simulink library "scp"  (R2021b)
settings: Solver=VariableStepAuto  StartTime=0.0  StopTime=10.0  RelTol=1e-3
undefined symbols (not defined in the file or in its folder): FALSE, KSCP_DelayECBAMandECDT_s, KSCP_DelayECDTandECDT_s, KSCP_DelayECDTandRCBAM_s, KSCP_DelayRCBAMandRCDT_s, KSCP_DelayRCDTandECBAM_s, KSCP_DelayRCDTandRCDT_s, KSCP_MCUMaxRefTq_Nm, TRUE
libraries: simulink x2
settings Model: Creator=FVT23118  LastModifiedBy=FVT23010

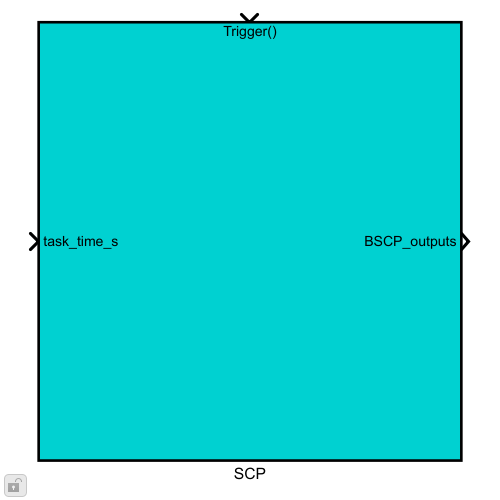
[thumbnail: Simulink's stored preview of the top-level diagram]
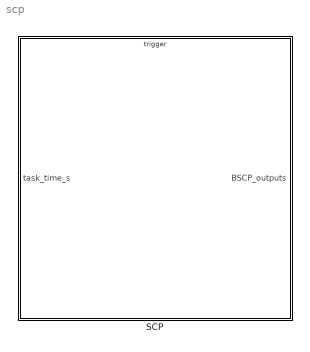
== system scp ==
  SCP : Subsystem

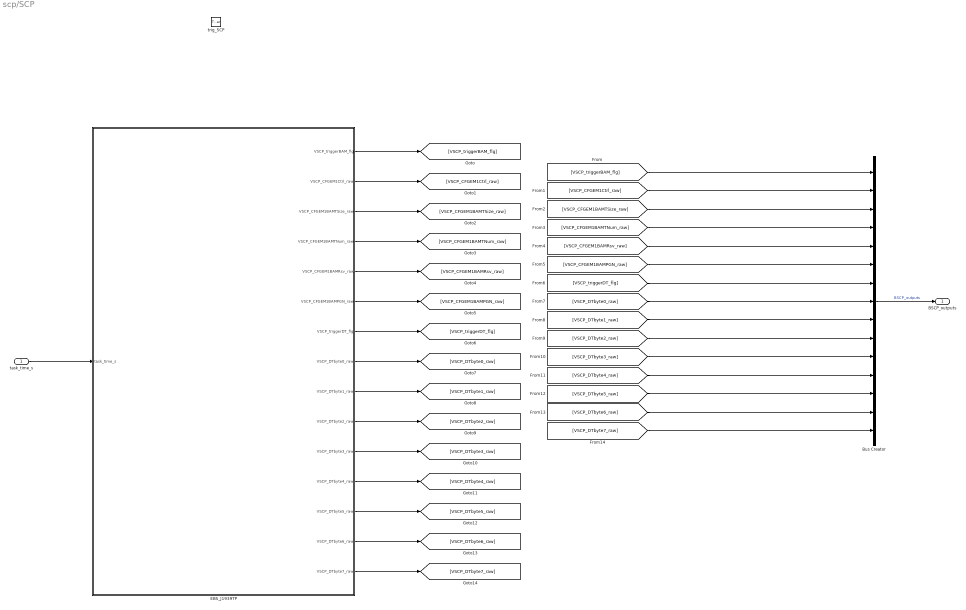
== system scp/SCP ==
  task_time_s : Inport
  trig_SCP : TriggerPort  TriggerType=function-call  VariantControl=(inherit)  PortDimensions=1
  Bus Creator : BusCreator  Inputs=15  OutDataTypeStr=Bus: BSCP_outputs  NonVirtualBus=on
  EBS_J1939TP : Subsystem
  BSCP_outputs : Outport  OutDataTypeStr=Bus: BSCP_outputs
  wires:
  Bus Creator/1 -> BSCP_outputs/1  "BSCP_outputs"
  EBS_J1939TP/5(VSCP_CFGEM1BAMRsv_raw) -> [VSCP_CFGEM1BAMRsv_raw]
  EBS_J1939TP/1(VSCP_triggerBAM_flg) -> [VSCP_triggerBAM_flg]
  task_time_s/1 -> EBS_J1939TP/1(task_time_s)
  EBS_J1939TP/2(VSCP_CFGEM1Ctrl_raw) -> [VSCP_CFGEM1Ctrl_raw]
  EBS_J1939TP/15(VSCP_DTbyte7_raw) -> [VSCP_DTbyte7_raw]
  EBS_J1939TP/14(VSCP_DTbyte6_raw) -> [VSCP_DTbyte6_raw]
  EBS_J1939TP/11(VSCP_DTbyte3_raw) -> [VSCP_DTbyte3_raw]
  EBS_J1939TP/9(VSCP_DTbyte1_raw) -> [VSCP_DTbyte1_raw]
  EBS_J1939TP/10(VSCP_DTbyte2_raw) -> [VSCP_DTbyte2_raw]
  EBS_J1939TP/7(VSCP_triggerDT_flg) -> [VSCP_triggerDT_flg]
  EBS_J1939TP/8(VSCP_DTbyte0_raw) -> [VSCP_DTbyte0_raw]
  EBS_J1939TP/6(VSCP_CFGEM1BAMPGN_raw) -> [VSCP_CFGEM1BAMPGN_raw]
  EBS_J1939TP/4(VSCP_CFGEM1BAMTNum_raw) -> [VSCP_CFGEM1BAMTNum_raw]
  EBS_J1939TP/13(VSCP_DTbyte5_raw) -> [VSCP_DTbyte5_raw]
  EBS_J1939TP/12(VSCP_DTbyte4_raw) -> [VSCP_DTbyte4_raw]
  EBS_J1939TP/3(VSCP_CFGEM1BAMTSize_raw) -> [VSCP_CFGEM1BAMTSize_raw]
  [VSCP_triggerBAM_flg] -> Bus Creator/1
  [VSCP_CFGEM1Ctrl_raw] -> Bus Creator/2
  [VSCP_CFGEM1BAMTSize_raw] -> Bus Creator/3
  [VSCP_CFGEM1BAMTNum_raw] -> Bus Creator/4
  [VSCP_CFGEM1BAMRsv_raw] -> Bus Creator/5
  [VSCP_CFGEM1BAMPGN_raw] -> Bus Creator/6
  [VSCP_triggerDT_flg] -> Bus Creator/7
  [VSCP_DTbyte0_raw] -> Bus Creator/8
  [VSCP_DTbyte1_raw] -> Bus Creator/9
  [VSCP_DTbyte2_raw] -> Bus Creator/10
  [VSCP_DTbyte3_raw] -> Bus Creator/11
  [VSCP_DTbyte4_raw] -> Bus Creator/12
  [VSCP_DTbyte5_raw] -> Bus Creator/13
  [VSCP_DTbyte6_raw] -> Bus Creator/14
  [VSCP_DTbyte7_raw] -> Bus Creator/15

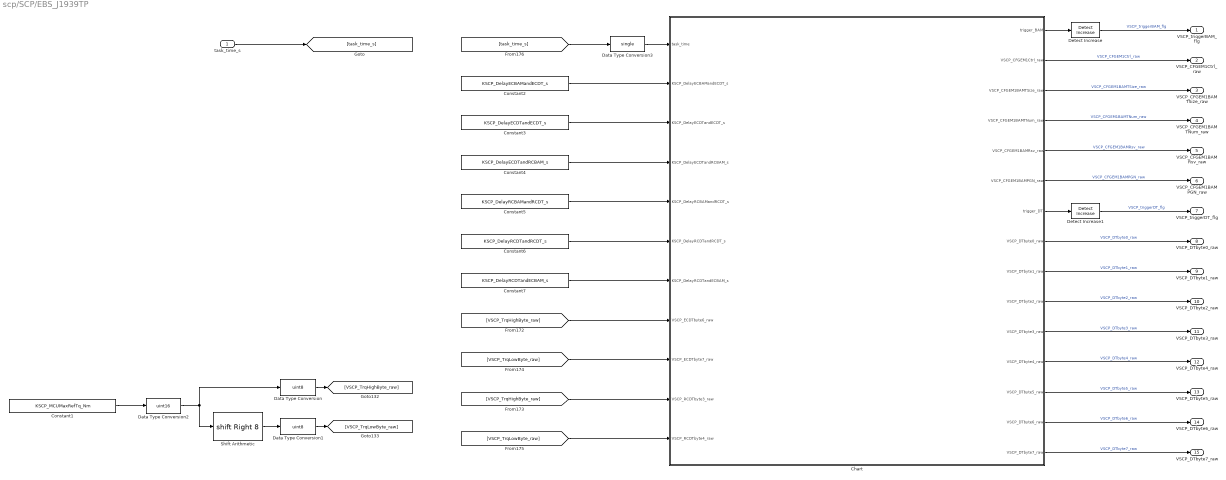
== system scp/SCP/EBS_J1939TP ==
  task_time_s : Inport
  Chart : Stateflow chart  TreatAsAtomicUnit=on
  Constant1 : Constant  Value=KSCP_MCUMaxRefTq_Nm
  Constant2 : Constant  Value=KSCP_DelayECBAMandECDT_s
  Constant3 : Constant  Value=KSCP_DelayECDTandECDT_s
  Constant4 : Constant  Value=KSCP_DelayECDTandRCBAM_s
  Constant5 : Constant  Value=KSCP_DelayRCBAMandRCDT_s
  Constant6 : Constant  Value=KSCP_DelayRCDTandRCDT_s
  Constant7 : Constant  Value=KSCP_DelayRCDTandECBAM_s
  Data Type Conversion : DataTypeConversion  OutDataTypeStr=uint8
  Data Type Conversion1 : DataTypeConversion  OutDataTypeStr=uint8
  Data Type Conversion2 : DataTypeConversion  OutDataTypeStr=uint16
  Data Type Conversion3 : DataTypeConversion  OutDataTypeStr=single
  Detect Increase : simulink/Logic and Bit Operations/Detect Increase  vinit=0.0  OutDataTypeStr=boolean
  Detect Increase1 : simulink/Logic and Bit Operations/Detect Increase  vinit=0.0  OutDataTypeStr=boolean
  Shift Arithmetic : ArithShift  BitShiftNumber=8  BitShiftDirection=Right
  VSCP_triggerBAM_flg : Outport
  VSCP_CFGEM1Ctrl_raw : Outport  Port=2
  VSCP_CFGEM1BAMTSize_raw : Outport  Port=3
  VSCP_CFGEM1BAMTNum_raw : Outport  Port=4
  VSCP_CFGEM1BAMRsv_raw : Outport  Port=5
  VSCP_CFGEM1BAMPGN_raw : Outport  Port=6
  VSCP_triggerDT_flg : Outport  Port=7
  VSCP_DTbyte0_raw : Outport  Port=8
  VSCP_DTbyte1_raw : Outport  Port=9
  VSCP_DTbyte2_raw : Outport  Port=10
  VSCP_DTbyte3_raw : Outport  Port=11
  VSCP_DTbyte4_raw : Outport  Port=12
  VSCP_DTbyte5_raw : Outport  Port=13
  VSCP_DTbyte6_raw : Outport  Port=14
  VSCP_DTbyte7_raw : Outport  Port=15
  wires:
  Data Type Conversion3/1 -> Chart/1(task_time)
  task_time_s/1 -> [task_time_s]
  Chart/15(VSCP_DTbyte7_raw) -> VSCP_DTbyte7_raw/1  "VSCP_DTbyte7_raw"
  Chart/14(VSCP_DTbyte6_raw) -> VSCP_DTbyte6_raw/1  "VSCP_DTbyte6_raw"
  Chart/13(VSCP_DTbyte5_raw) -> VSCP_DTbyte5_raw/1  "VSCP_DTbyte5_raw"
  Chart/12(VSCP_DTbyte4_raw) -> VSCP_DTbyte4_raw/1  "VSCP_DTbyte4_raw"
  Chart/11(VSCP_DTbyte3_raw) -> VSCP_DTbyte3_raw/1  "VSCP_DTbyte3_raw"
  Chart/10(VSCP_DTbyte2_raw) -> VSCP_DTbyte2_raw/1  "VSCP_DTbyte2_raw"
  Chart/9(VSCP_DTbyte1_raw) -> VSCP_DTbyte1_raw/1  "VSCP_DTbyte1_raw"
  Chart/8(VSCP_DTbyte0_raw) -> VSCP_DTbyte0_raw/1  "VSCP_DTbyte0_raw"
  Detect Increase1/1 -> VSCP_triggerDT_flg/1  "VSCP_triggerDT_flg"
  Chart/6(VSCP_CFGEM1BAMPGN_raw) -> VSCP_CFGEM1BAMPGN_raw/1  "VSCP_CFGEM1BAMPGN_raw"
  Chart/5(VSCP_CFGEM1BAMRsv_raw) -> VSCP_CFGEM1BAMRsv_raw/1  "VSCP_CFGEM1BAMRsv_raw"
  Chart/4(VSCP_CFGEM1BAMTNum_raw) -> VSCP_CFGEM1BAMTNum_raw/1  "VSCP_CFGEM1BAMTNum_raw"
  Chart/3(VSCP_CFGEM1BAMTSize_raw) -> VSCP_CFGEM1BAMTSize_raw/1  "VSCP_CFGEM1BAMTSize_raw"
  Chart/2(VSCP_CFGEM1Ctrl_raw) -> VSCP_CFGEM1Ctrl_raw/1  "VSCP_CFGEM1Ctrl_raw"
  Detect Increase/1 -> VSCP_triggerBAM_flg/1  "VSCP_triggerBAM_flg"
  Chart/7(trigger_DT) -> Detect Increase1/1
  Chart/1(trigger_BAM) -> Detect Increase/1
  Constant7/1 -> Chart/7(KSCP_DelayRCDTandECBAM_s)
  [VSCP_TrqLowByte_raw] -> Chart/9(VSCP_ECDTbyte7_raw)
  Data Type Conversion/1 -> [VSCP_TrqHighByte_raw]
  Constant6/1 -> Chart/6(KSCP_DelayRCDTandRCDT_s)
  Constant3/1 -> Chart/3(KSCP_DelayECDTandECDT_s)
  Shift Arithmetic/1 -> Data Type Conversion1/1
  Data Type Conversion2/1 -> Shift Arithmetic/1, Data Type Conversion/1
  Constant5/1 -> Chart/5(KSCP_DelayRCBAMandRCDT_s)
  Constant1/1 -> Data Type Conversion2/1
  [VSCP_TrqLowByte_raw] -> Chart/11(VSCP_RCDTbyte4_raw)
  Constant4/1 -> Chart/4(KSCP_DelayECDTandRCBAM_s)
  [VSCP_TrqHighByte_raw] -> Chart/8(VSCP_ECDTbyte6_raw)
  [VSCP_TrqHighByte_raw] -> Chart/10(VSCP_RCDTbyte3_raw)
  Data Type Conversion1/1 -> [VSCP_TrqLowByte_raw]
  [task_time_s] -> Data Type Conversion3/1
  Constant2/1 -> Chart/2(KSCP_DelayECBAMandECDT_s)

== stateflow chart scp/SCP/EBS_J1939TP/Chart ==
  state TP
    state Trigger_ECBAM_and_Delay
      en: trigger_BAM = TRUE;
      (default) -> (junction 21) : {
          |  VSCP_TpDelayDone_flg = FALSE;
          |  VSCP_TimeTPdelay_s = 0;
          | }
      Trigger_ECBAM_and_Delay -> (junction 21) [order 1] : {trigger_BAM = FALSE;}
      (junction 21) -> (junction 26) [order 1] : [VSCP_TimeTPdelay_s >= KSCP_DelayECBAMandECDT_s]
      (junction 21) -> (junction 24) [order 2] : {VSCP_TimeTPdelay_s += task_time;}
      (junction 26) -> (junction 28) : {VSCP_TpDelayDone_flg = TRUE;}
      (junction 28) -> (junction 24)
    state Tirgger_ECDT1_and_Delay
      en: trigger_DT = TRUE;
      (default) -> (junction 32) : {
          |  VSCP_TpDelayDone_flg = FALSE;
          |  VSCP_TimeTPdelay_s = 0;}
      Tirgger_ECDT1_and_Delay -> (junction 32) [order 1] : {trigger_DT = FALSE;}
      (junction 32) -> (junction 33) [order 1] : [VSCP_TimeTPdelay_s >= KSCP_DelayECDTandECDT_s]
      (junction 32) -> (junction 34) [order 2] : {VSCP_TimeTPdelay_s += task_time;}
      (junction 33) -> (junction 35) : {VSCP_TpDelayDone_flg = TRUE;}
      (junction 35) -> (junction 34)
    state Tirgger_ECDT2_and_Delay
      en: trigger_DT = TRUE;
      (default) -> (junction 55) : {
          |  VSCP_TpDelayDone_flg = FALSE;
          |  VSCP_TimeTPdelay_s = 0;}
      Tirgger_ECDT2_and_Delay -> (junction 55) [order 1] : {trigger_DT = FALSE;}
      (junction 55) -> (junction 56) [order 1] : [VSCP_TimeTPdelay_s >= KSCP_DelayECDTandECDT_s]
      (junction 55) -> (junction 57) [order 2] : {VSCP_TimeTPdelay_s += task_time;}
      (junction 56) -> (junction 58) : {VSCP_TpDelayDone_flg = TRUE;}
      (junction 58) -> (junction 57)
    state Tirgger_ECDT3_and_Delay
      en: trigger_DT = TRUE;
      (default) -> (junction 123) : {
          |  VSCP_TpDelayDone_flg = FALSE;
          |  VSCP_TimeTPdelay_s = 0;}
      Tirgger_ECDT3_and_Delay -> (junction 123) [order 1] : {trigger_DT = FALSE;}
      (junction 123) -> (junction 124) [order 1] : [VSCP_TimeTPdelay_s >= KSCP_DelayECDTandECDT_s]
      (junction 123) -> (junction 125) [order 2] : {VSCP_TimeTPdelay_s += task_time;}
      (junction 124) -> (junction 126) : {VSCP_TpDelayDone_flg = TRUE;}
      (junction 126) -> (junction 125)
    state Tirgger_ECDT4_and_Delay
      en: trigger_DT = TRUE;
      (default) -> (junction 134) : {
          |  VSCP_TpDelayDone_flg = FALSE;
          |  VSCP_TimeTPdelay_s = 0;}
      Tirgger_ECDT4_and_Delay -> (junction 134) [order 1] : {trigger_DT = FALSE;}
      (junction 134) -> (junction 135) [order 1] : [VSCP_TimeTPdelay_s >= KSCP_DelayECDTandECDT_s]
      (junction 134) -> (junction 136) [order 2] : {VSCP_TimeTPdelay_s += task_time;}
      (junction 135) -> (junction 137) : {VSCP_TpDelayDone_flg = TRUE;}
      (junction 137) -> (junction 136)
    state Tirgger_ECDT5_and_Delay
      en: trigger_DT = TRUE;
      (default) -> (junction 145) : {
          |  VSCP_TpDelayDone_flg = FALSE;
          |  VSCP_TimeTPdelay_s = 0;}
      Tirgger_ECDT5_and_Delay -> (junction 145) [order 1] : {trigger_DT = FALSE;}
      (junction 145) -> (junction 146) [order 1] : [VSCP_TimeTPdelay_s >= KSCP_DelayECDTandECDT_s]
      (junction 145) -> (junction 147) [order 2] : {VSCP_TimeTPdelay_s += task_time;}
      (junction 146) -> (junction 148) : {VSCP_TpDelayDone_flg = TRUE;}
      (junction 148) -> (junction 147)
    state Tirgger_ECDT6_and_Delay
      en: trigger_DT = TRUE;
      (default) -> (junction 156) : {
          |  VSCP_TpDelayDone_flg = FALSE;
          |  VSCP_TimeTPdelay_s = 0;}
      Tirgger_ECDT6_and_Delay -> (junction 156) [order 1] : {trigger_DT = FALSE;}
      (junction 156) -> (junction 157) [order 1] : [VSCP_TimeTPdelay_s >= KSCP_DelayECDTandRCBAM_s]
      (junction 156) -> (junction 158) [order 2] : {VSCP_TimeTPdelay_s += task_time;}
      (junction 157) -> (junction 159) : {VSCP_TpDelayDone_flg = TRUE;}
      (junction 159) -> (junction 158)
    state Trigger_RCBAM_and_Delay
      en: trigger_BAM = TRUE;
      (default) -> (junction 67) : {
          |  VSCP_TpDelayDone_flg = FALSE;
          |  VSCP_TimeTPdelay_s = 0;}
      Trigger_RCBAM_and_Delay -> (junction 67) [order 1] : {trigger_BAM = FALSE;}
      (junction 67) -> (junction 68) [order 1] : [VSCP_TimeTPdelay_s >= KSCP_DelayRCBAMandRCDT_s]
      (junction 67) -> (junction 69) [order 2] : {VSCP_TimeTPdelay_s += task_time;}
      (junction 68) -> (junction 70) : {VSCP_TpDelayDone_flg = TRUE;}
      (junction 70) -> (junction 69)
    state Tirgger_RCDT1_and_Delay
      en: trigger_DT = TRUE;
      (default) -> (junction 79) : {
          |  VSCP_TpDelayDone_flg = FALSE;
          |  VSCP_TimeTPdelay_s = 0;}
      Tirgger_RCDT1_and_Delay -> (junction 79) [order 1] : {trigger_DT = FALSE;}
      (junction 79) -> (junction 80) [order 1] : [VSCP_TimeTPdelay_s >= KSCP_DelayRCDTandRCDT_s]
      (junction 79) -> (junction 81) [order 2] : {VSCP_TimeTPdelay_s += task_time;}
      (junction 80) -> (junction 82) : {VSCP_TpDelayDone_flg = TRUE;}
      (junction 82) -> (junction 81)
    state Tirgger_RCDT2_and_Delay
      en: trigger_DT = TRUE;
      (default) -> (junction 300) : {
          |  VSCP_TpDelayDone_flg = FALSE;
          |  VSCP_TimeTPdelay_s = 0;}
      Tirgger_RCDT2_and_Delay -> (junction 300) [order 1] : {trigger_DT = FALSE;}
      (junction 300) -> (junction 301) [order 1] : [VSCP_TimeTPdelay_s >= KSCP_DelayRCDTandRCDT_s]
      (junction 300) -> (junction 302) [order 2] : {VSCP_TimeTPdelay_s += task_time;}
      (junction 301) -> (junction 303) : {VSCP_TpDelayDone_flg = TRUE;}
      (junction 303) -> (junction 302)
    state Tirgger_RCDT3_and_Delay
      en: trigger_DT = TRUE;
      (default) -> (junction 311) : {
          |  VSCP_TpDelayDone_flg = FALSE;
          |  VSCP_TimeTPdelay_s = 0;}
      Tirgger_RCDT3_and_Delay -> (junction 311) [order 1] : {trigger_DT = FALSE;}
      (junction 311) -> (junction 312) [order 1] : [VSCP_TimeTPdelay_s >= KSCP_DelayRCDTandECBAM_s]
      (junction 311) -> (junction 313) [order 2] : {VSCP_TimeTPdelay_s += task_time;}
      (junction 312) -> (junction 314) : {VSCP_TpDelayDone_flg = TRUE;}
      (junction 314) -> (junction 313)
    (default) -> (junction 3)
    (junction 119) -> (junction 3)
    (junction 117) -> (junction 119)
    (junction 3) -> Trigger_ECBAM_and_Delay : { VSCP_CFGEM1Ctrl_raw = 0x20;
        |   VSCP_CFGEM1BAMTSize_raw = 0x27;
        |   VSCP_CFGEM1BAMTNum_raw = 0x06;
        |   VSCP_CFGEM1BAMRsv_raw = 0xFF;
        |   VSCP_CFGEM1BAMPGN_raw = 0xFEE3;}
    Trigger_ECBAM_and_Delay -> Tirgger_ECDT1_and_Delay [order 1] : [VSCP_TpDelayDone_flg]
        | {VSCP_DTbyte0_raw = 0x01; VSCP_DTbyte1_raw = 0xFF; VSCP_DTbyte2_raw = 0xFF; VSCP_DTbyte3_raw = 0xFF;
        |  VSCP_DTbyte4_raw = 0xFF; VSCP_DTbyte5_raw = 0xFF; VSCP_DTbyte6_raw = 0xFF; VSCP_DTbyte7_raw = 0xFF;}
    Tirgger_ECDT1_and_Delay -> Tirgger_ECDT2_and_Delay [order 1] : [VSCP_TpDelayDone_flg]
        | {VSCP_DTbyte0_raw = 0x02; VSCP_DTbyte1_raw = 0xFF; VSCP_DTbyte2_raw = 0xFF; VSCP_DTbyte3_raw = 0xFF;
        |  VSCP_DTbyte4_raw = 0xFF; VSCP_DTbyte5_raw = 0xFF; VSCP_DTbyte6_raw = 0xFF; VSCP_DTbyte7_raw = 0xFF;}
    Tirgger_ECDT2_and_Delay -> Tirgger_ECDT3_and_Delay [order 1] : [VSCP_TpDelayDone_flg]
        | {VSCP_DTbyte0_raw = 0x03; VSCP_DTbyte1_raw = 0xFF; VSCP_DTbyte2_raw = 0xFF; VSCP_DTbyte3_raw = 0xFF;
        |  VSCP_DTbyte4_raw = 0xFF; VSCP_DTbyte5_raw = 0xFF; VSCP_DTbyte6_raw = VSCP_ECDTbyte6_raw; VSCP_DTbyte7_raw = VSCP_ECDTbyte7_raw;}
    Tirgger_ECDT3_and_Delay -> Tirgger_ECDT4_and_Delay [order 1] : [VSCP_TpDelayDone_flg]
        | {VSCP_DTbyte0_raw = 0x04; VSCP_DTbyte1_raw = 0xFF; VSCP_DTbyte2_raw = 0xFF; VSCP_DTbyte3_raw = 0xFF;
        |  VSCP_DTbyte4_raw = 0xFF; VSCP_DTbyte5_raw = 0xFF; VSCP_DTbyte6_raw = 0xFF; VSCP_DTbyte7_raw = 0xFF;}
    Tirgger_ECDT4_and_Delay -> Tirgger_ECDT5_and_Delay [order 1] : [VSCP_TpDelayDone_flg]
        | {VSCP_DTbyte0_raw = 0x05; VSCP_DTbyte1_raw = 0xFF; VSCP_DTbyte2_raw = 0xFF; VSCP_DTbyte3_raw = 0xFF;
        |  VSCP_DTbyte4_raw = 0xFF; VSCP_DTbyte5_raw = 0xFF; VSCP_DTbyte6_raw = 0xFF; VSCP_DTbyte7_raw = 0xFF;}
    Tirgger_ECDT5_and_Delay -> Tirgger_ECDT6_and_Delay [order 1] : [VSCP_TpDelayDone_flg]
        | {VSCP_DTbyte0_raw = 0x06; VSCP_DTbyte1_raw = 0xFF; VSCP_DTbyte2_raw = 0xFF; VSCP_DTbyte3_raw = 0xFF;
        |  VSCP_DTbyte4_raw = 0xFF; VSCP_DTbyte5_raw = 0xFF; VSCP_DTbyte6_raw = 0xFF; VSCP_DTbyte7_raw = 0xFF;}
    Tirgger_ECDT6_and_Delay -> Trigger_RCBAM_and_Delay [order 1] : [VSCP_TpDelayDone_flg]
        | { VSCP_CFGEM1Ctrl_raw = 0x20;
        |   VSCP_CFGEM1BAMTSize_raw = 0x13;
        |   VSCP_CFGEM1BAMTNum_raw = 0x03;
        |   VSCP_CFGEM1BAMRsv_raw = 0xFF;
        |   VSCP_CFGEM1BAMPGN_raw = 0xFEE1;}
    Trigger_RCBAM_and_Delay -> Tirgger_RCDT1_and_Delay [order 1] : [VSCP_TpDelayDone_flg]
        | {VSCP_DTbyte0_raw = 0x01; VSCP_DTbyte1_raw = 0x40; VSCP_DTbyte2_raw = 0xFF; VSCP_DTbyte3_raw = 0xFF;
        |  VSCP_DTbyte4_raw = 0xFF; VSCP_DTbyte5_raw = 0xFF; VSCP_DTbyte6_raw = 0xFF; VSCP_DTbyte7_raw = 0xFF;}
    Tirgger_RCDT1_and_Delay -> Tirgger_RCDT2_and_Delay [order 1] : [VSCP_TpDelayDone_flg]
        | {VSCP_DTbyte0_raw = 0x02; VSCP_DTbyte1_raw = 0xFF; VSCP_DTbyte2_raw = 0xFF; VSCP_DTbyte3_raw = 0xFF;
        |  VSCP_DTbyte4_raw = 0xFF; VSCP_DTbyte5_raw = 0xFF; VSCP_DTbyte6_raw = 0xFF; VSCP_DTbyte7_raw = 0xFF;}
    Tirgger_RCDT2_and_Delay -> Tirgger_RCDT3_and_Delay [order 1] : [VSCP_TpDelayDone_flg]
        | {VSCP_DTbyte0_raw = 0x03; VSCP_DTbyte1_raw = 0xFF; VSCP_DTbyte2_raw = 0xFF; VSCP_DTbyte3_raw = VSCP_RCDTbyte3_raw;
        |  VSCP_DTbyte4_raw = VSCP_RCDTbyte4_raw; VSCP_DTbyte5_raw = 0xFF; VSCP_DTbyte6_raw = 0xFF; VSCP_DTbyte7_raw = 0xFF;}
    Tirgger_RCDT3_and_Delay -> (junction 115) [order 1] : [VSCP_TpDelayDone_flg]
    (junction 115) -> (junction 117)
  (default) -> TP
  data: task_time input; KSCP_DelayECBAMandECDT_s input; KSCP_DelayECDTandECDT_s input; KSCP_DelayECDTandRCBAM_s input; trigger_BAM output boolean; VSCP_CFGEM1Ctrl_raw output uint8; VSCP_CFGEM1BAMTSize_raw output uint16; VSCP_CFGEM1BAMTNum_raw output uint8; VSCP_CFGEM1BAMRsv_raw output uint8; VSCP_CFGEM1BAMPGN_raw output uint32; trigger_DT output boolean; VSCP_TimeTPdelay_s local single; TRUE parameter; FALSE parameter; VSCP_TpDelayDone_flg local boolean; KSCP_DelayRCBAMandRCDT_s input; KSCP_DelayRCDTandRCDT_s input; KSCP_DelayRCDTandECBAM_s input; VSCP_DTbyte0_raw output uint8; VSCP_DTbyte1_raw output uint8; VSCP_DTbyte2_raw output uint8; VSCP_DTbyte3_raw output uint8; VSCP_DTbyte4_raw output uint8; VSCP_DTbyte5_raw output uint8; VSCP_DTbyte6_raw output uint8; VSCP_DTbyte7_raw output uint8; VSCP_ECDTbyte6_raw input; VSCP_ECDTbyte7_raw input; VSCP_RCDTbyte3_raw input; VSCP_RCDTbyte4_raw input
